simulink model "fuzblock"  (Simulink 2.20)
settings: Solver=ode45  StartTime=0  StopTime=10000  MaxStep=0.1  RelTol=1e-3  AbsTol=1e-6
settings Model: SaveTime=off  SaveOutput=off  ConsistencyChecking=off  RTWPlaceOutputsASAP=off  RTWTemplateMakefile=grt_unix.tmf

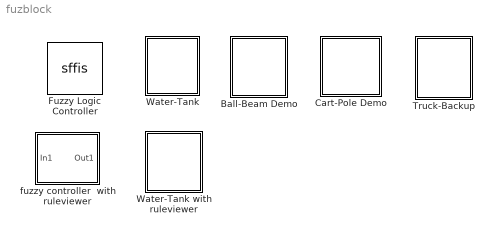
== system fuzblock ==
  Ball-Beam Demo : Subsystem
      settings: OpenFcn=slbb
  Cart-Pole Demo : Subsystem
      settings: OpenFcn=slcp
  Fuzzy Logic Controller : S-Function  FunctionName=sffis  Parameters=fismatrix  PortCounts=[]  SFunctionModules=sfsup  mask(FIS){@1=fismat}
      mask prompts: @1 "FIS Matrix:"
      mask help: FIS
      mask init:
      | fismatrix = @1;
      mask Help: Fuzzy Inference System
      mask Display: plot(0, -0.3, 6, -0.3, 0, 1.2, 6, 1.2, [0 6], [0 0], [1 2 3],[0 1 0],[2 3 4],[0 1 0],[3 4 5],[0 1 0])
  Truck-Backup : Subsystem
      settings: OpenFcn=sltbu
  Water-Tank : Subsystem
      settings: OpenFcn=sltank
  Water-Tank with ruleviewer : Subsystem
      settings: OpenFcn=sltankrule
  fuzzy controller  with ruleviewer : Subsystem
      mask Type: FIS
      mask Display: plot(0, -0.3, 6, -0.3, 0, 1.2, 6, 1.2, [0 6], [0 0], [1 2 3],[0 1 0],[2 3 4],[0 1 0],[3 4 5],[0 1 0])

== system fuzblock/Ball-Beam Demo ==

== system fuzblock/Cart-Pole Demo ==

== system fuzblock/Truck-Backup ==

== system fuzblock/Water-Tank ==

== system fuzblock/Water-Tank with ruleviewer ==

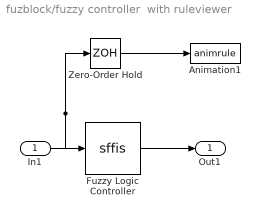
== system fuzblock/fuzzy controller  with ruleviewer ==
  In1 : Inport  Port=1  PortWidth=-1  SampleTime=-1
  Animation1 : S-Function  FunctionName=animrule  Parameters=fismatrix  PortCounts=[]  SFunctionModules=''
  Fuzzy Logic Controller : S-Function  FunctionName=sffis  Parameters=fismatrix  PortCounts=[]  SFunctionModules=sfsup  mask(FIS){@1=fismat}
      mask prompts: @1 "FIS Matrix:"
      mask help: FIS
      mask init:
      | fismatrix = @1;
      mask Help: Fuzzy Inference System
      mask Display: plot(0, -0.3, 6, -0.3, 0, 1.2, 6, 1.2, [0 6], [0 0], [1 2 3],[0 1 0],[2 3 4],[0 1 0],[3 4 5],[0 1 0])
  Zero-Order Hold : ZeroOrderHold  SampleTime=2
  Out1 : Outport  Port=1  InitialOutput=0
  wires:
  Zero-Order Hold/1 -> Animation1/1
  Fuzzy Logic Controller/1 -> Out1/1
  In1/1 -> Zero-Order Hold/1, Fuzzy Logic Controller/1
